simulink library "flowInterp_ul"  (R2018b)
settings: Solver=VariableStepAuto  StartTime=0.0  StopTime=10.0  RelTol=1e-3
values from neighbouring files (symbols this model uses):
  heights = timeseries(repmat(heights,1,1,2),[0 simTime])    [BAT_ts.m]    (also in environment.m = heights(:))
undefined symbols (not defined in the file or in its folder): Flow
libraries: simulink x1
settings Model: Creator=Ayaz  LastModifiedBy=Ayaz

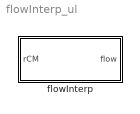
== system flowInterp_ul ==
  flowInterp : Subsystem  mask{altiVals=heights, flowVals=Flow}
      mask prompts: altiVals "Altitude values"; flowVals "Flow values"

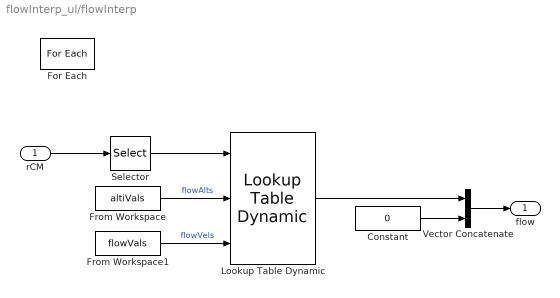
== system flowInterp_ul/flowInterp ==
  rCM : Inport  Partition=on  PartitionDimension=2  PartitionWidth=1  PartitionOffset=0
  Constant : Constant  Value=0
  For Each : ForEach  DisableCoverage=on  IndexMode=One-based
  From Workspace : FromWorkspace  VariableName=altiVals  SampleTime=0  OutputAfterFinalValue=Holding final value
  From Workspace1 : FromWorkspace  VariableName=flowVals  SampleTime=0  OutputAfterFinalValue=Holding final value
  Lookup Table Dynamic : simulink/Lookup Tables/Lookup Table Dynamic  LookUpMeth=Interpolation-Use End Values  OutDataType=fixdt('double')  OutScaling=[]  OutputDataTypeScalingMode=Specify via dialog  OutDataTypeStr=double  DoSatur=off
      settings: SourceProductName=Simulink
  Selector : Selector  InputPortWidth=2  IndexOptions=Index vector (dialog)  Indices=2  OutputSizes=1
  Vector Concatenate : Concatenate
  flow : Outport  ConcatenationDimension=2
  wires:
  rCM/1 -> Selector/1
  Lookup Table Dynamic/1 -> Vector Concatenate/1
  From Workspace/1 -> Lookup Table Dynamic/2  "flowAlts"
  From Workspace1/1 -> Lookup Table Dynamic/3  "flowVels"
  Selector/1 -> Lookup Table Dynamic/1
  Constant/1 -> Vector Concatenate/2
  Vector Concatenate/1 -> flow/1
